simulink model "DOC_Model"  (R2019a)
settings: Solver=VariableStepAuto  StartTime=0.0  StopTime=10.0  RelTol=1e-3
libraries: simulink x2
settings Model: DataDictionary=DOC_Model_DD.sldd  Creator=Kore  LastModifiedBy=Kore

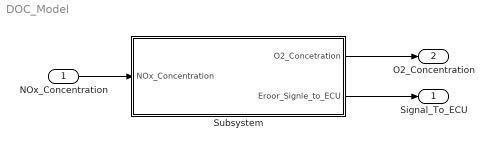
== system DOC_Model ==
  NOx_Concentration : Inport
  Subsystem : Subsystem
  Signal_To_ECU : Outport
  O2_Concentration : Outport  Port=2
  wires:
  Subsystem/2(Eroor_Signle_to_ECU) -> Signal_To_ECU/1
  Subsystem/1(O2_Concetration) -> O2_Concentration/1
  NOx_Concentration/1 -> Subsystem/1(NOx_Concentration)

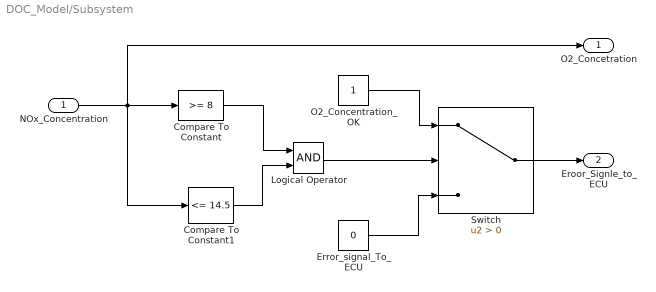
== system DOC_Model/Subsystem ==
  NOx_Concentration : Inport
  Compare To Constant : simulink/Logic and Bit Operations/Compare To Constant  relop=>=  const=8  OutDataTypeStr=boolean
  Compare To Constant1 : simulink/Logic and Bit Operations/Compare To Constant  relop=<=  const=14.5  OutDataTypeStr=boolean
  "Error_signal_To_ECU " : Constant  Value=0
  Logical Operator : Logic  AllPortsSameDT=off  OutDataTypeStr=boolean
  O2_Concentration_OK : Constant
  Switch : Switch  Criteria=u2 > Threshold
  O2_Concetration : Outport
  Eroor_Signle_to_ECU : Outport  Port=2
  wires:
  Compare To Constant/1 -> Logical Operator/1
  Logical Operator/1 -> Switch/2
  NOx_Concentration/1 -> O2_Concetration/1, Compare To Constant1/1, Compare To Constant/1
  "Error_signal_To_ECU "/1 -> Switch/3
  O2_Concentration_OK/1 -> Switch/1
  Compare To Constant1/1 -> Logical Operator/2
  Switch/1 -> Eroor_Signle_to_ECU/1
